simulink model "state_space"  (R2018b)
settings: Solver=VariableStepAuto  StartTime=0.0  StopTime=10.0  RelTol=1e-3
values from neighbouring files (symbols this model uses):
  K_delay = place(sys_discrete.A, sys_discrete.B, discrete_poles)    [pole_placement_delay.m]
settings Model: Creator=lorenzoterenzi  LastModifiedBy=lorenzoterenzi

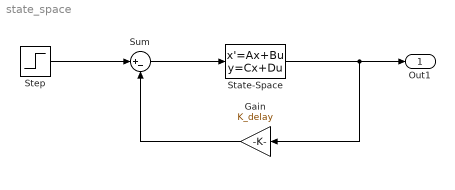
== system state_space ==
  Gain : Gain  Gain=K_delay
  State-Space : StateSpace  InitialCondition=0
  Step : Step  SampleTime=0
  Sum : Sum  Inputs=|+-
  Out1 : Outport
  wires:
  Step/1 -> Sum/1
  Sum/1 -> State-Space/1
  Gain/1 -> Sum/2
  State-Space/1 -> Gain/1, Out1/1
